simulink model "trabalho_freq_fourier"  (R2015a)
settings: Solver=ode45  StartTime=0.0  StopTime=10.0  RelTol=1e-3
libraries: simulink x1
settings Model: Creator=Roberto  LastModifiedBy=Roberto

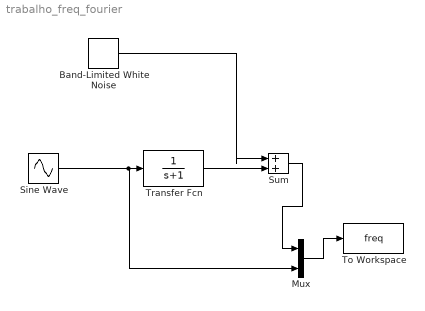
== system trabalho_freq_fourier ==
  Band-Limited White Noise : simulink/Sources/Band-Limited White Noise  Cov=[0.1]  Ts=0.1  seed=[23341]
  Mux : Mux  Inputs=2
  Sine Wave : Sin  SampleTime=0
  Sum : Sum  Inputs=|++
  To Workspace : ToWorkspace  VariableName=freq  SampleTime=-1
  Transfer Fcn : TransferFcn  Denominator=[1 1]
  wires:
  Transfer Fcn/1 -> Sum/2
  Band-Limited White Noise/1 -> Sum/1
  Sine Wave/1 -> Mux/2, Transfer Fcn/1
  Mux/1 -> To Workspace/1
  Sum/1 -> Mux/1
